simulink model "CAVE_MachE_speedTrack0202"  (R2019b)
settings: configuration reference "ConfigSetDesktopFixedStep" (kept outside this file)
PreLoadFcn:
  | VSS_BICYCLE=Simulink.Variant('Dual=0');
  | VSS_DUAL=Simulink.Variant('Dual=1');
  | Dual=1;
  | load('DriveCycle2.mat')
PostLoadFcn:
  | if any(exist('dsrtsu_mdlpostloadfcn', 'file') ~= 0), dsrtsu_mdlpostloadfcn('Execute', bdroot); end
InitFcn:
  | , if any(exist('dsmpb_private', 'file') ~= 0), dsmpb_private('dsmpb_mdlclblib', 'Init', bdroot); end,
  | load('DriveCycle2.mat')
model workspace (MAT data in the model file):
  Gas = 0.383333333333
values from neighbouring files (symbols this model uses):
  CoastDown =     [Run_Simulink.mat]
  limitedMCT =     [Run_Simulink.mat]
  MCT =     [Run_Simulink.mat]
  pMCT =     [Run_Simulink.mat]
  Ref_speed = [13 13.007895099 13.015778396 13.023649891 13.031509584 13.039357475 13.047193564 13.055017851 13.062830336 13.070631019 13.0784199 13.086196979 ... (2669 elements, 2669x1)]    [Ref_speed_and_time.mat]
  Ref_time = [0 0.01 0.02 0.03 0.04 0.05 0.06 0.07 0.08 0.09 0.1 0.11 ... (2669 elements, 2669x1)]    [Ref_speed_and_time.mat]
  US06 =     [Run_Simulink.mat]
undefined symbols (not defined in the file or in its folder): AccelCmd, ActTqLF_Nm_, ActTqLR_Nm_, ActTqRF_Nm_, ActTqRR_Nm_, BattChargeLimitMaxPwr, BattChargeLimitSocBpts, BattChargeLimitTbl, BattChrgCapcty, BattDischargeLimitSocBpts, BattDischargeLimitTbl, BattDischargeMaxPwr, BattNumCellsParallel, BattNumCellsSeries, BattOpenVoltCapBpts, BattOpenVoltTbl, BattResistSocBpts, BattResistTbl, BattResistTempBpts, BrakeMaxPrs, BrakeMaxTrq, ChassisDistCg2FrontAxle, ChassisDistCg2RearAxle, ChassisVehMass, CltchCmd, DecelCmd, DiffRatio, DiscIntNeverNeededParam, EnvGravCnst, EnvPrs, EnvTemp, FuelSpecificGrav, GearCmd, h, InitStates, lgSw, MtrEffSpdBpts, MtrEffTbl, MtrEffTrqBpts, MtrPwrMax, MtrTrqMax, Ref_Spd0229, Ref_Time0229, SteeringCmd, SupvsryCtrlRegenBrkCutOffTbl, SupvsryCtrlRegenSpdBpts, TestScnrioCycleNum, VEH
libraries: VSIGenLib x67, simulink x57, etargetslib x38, dsmpblib x28, vehdynlibtire x12, autolibshared x9, vehdynlibsuspension x7, vehdynlibtirecommon x7, autolibutils x5, CarMaker4SL x4, VsrLibWheel x4, autolibpowerinfoutils x3
(part 13 of 14)

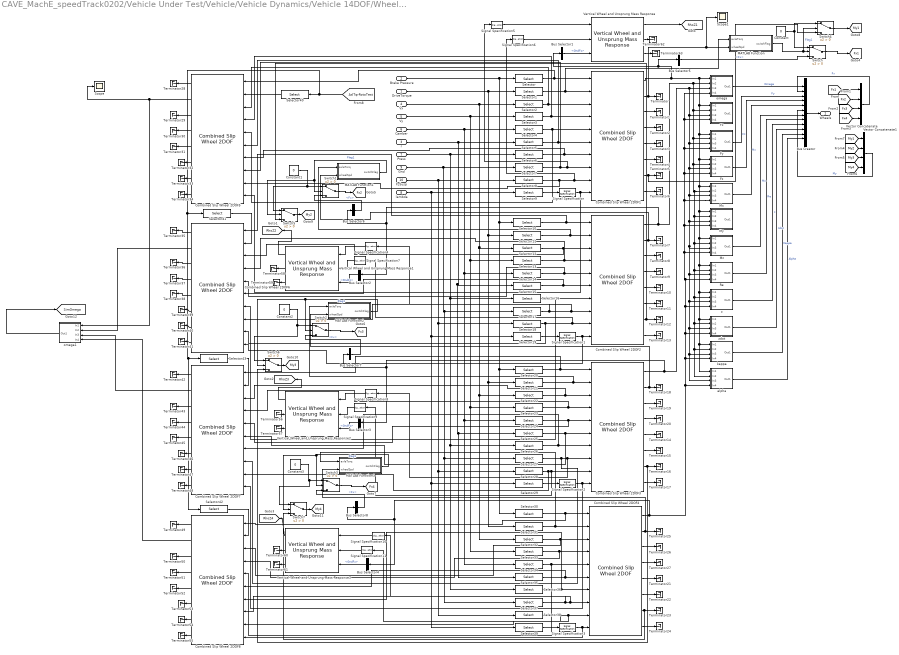
== system CAVE_MachE_speedTrack0202/Vehicle Under Test/Vehicle/Vehicle Dynamics/Vehicle 14DOF/Wheels and Tires/VDBS/Tires/MF Tires ==
  DriveTorque : Inport
  Brake Pressure : Inport  Port=2
  r : Inport  Port=3
  Vx : Inport  Port=4
  Vy : Inport  Port=5
  Camber : Inport  Port=6
  Press : Inport  Port=7  Unit=Pa
  lambda : Inport  Port=8  Unit=1
  Gnd : Inport  Port=9
  FzSusp : Inport  Port=10
  Bus Creator : BusCreator  Inputs=12
  Bus Selector{1..4} (4 alike) : BusSelector  OutputSignals=GndFz
  Bus Selector{5..8} (4 alike) : BusSelector  OutputSignals=Fx
  Combined Slip Wheel 2DOF{1..8} (8 alike) : vehdynlibtire/Combined Slip Wheel 2DOF  BrakeType=Disc  mu_static=.3  mu_kinetic=.2  disk_abore=.05  Rm=.216  num_pads=4  drum_abore=0.0508  drum_a=0.123  drum_c=0.212  drum_r=0.15  drum_theta1=0  drum_theta2=126  brake_p_bpt=[0 BrakeMaxPrs]/1e5  brake_n_bpt=[0 1000]  f_brake_t=[0 0; BrakeMaxTrq BrakeMaxTrq ]  tireParamSet=vdynPassCar.mat  plySteer=off  turnslip=off  PRESMAX=1000000  PRESMIN=10000  FZMAX=10000  FZMIN=100  VXLOW=0.1  KPUMAX=1.5  KPUMIN=-1.5  ALPMAX=1.5  ALPMIN=-1.5  CAMMAX=0.2  CAMMIN=-0.2  LONGVL=16.7  omegao=0  br=1e-3  UNLOADED_RADIUS=0.3135  NOMPRES=220000  FNOMIN=5000  WIDTH=0.235  MASS=13.37  IYY=0.82  GRAVITY=-9.81  zo=.015+0  zdoto=0  BREFF=8.25094594147963  DREFF=0.260468730454265  FREFF=0.0735298544471851  Q_RE0=1.00866439868088  Q_V1=0.000760413786224011  Q_V2=0.0463384792019201  Q_FZ1=0  Q_FZ2=15.6870832810226  Q_FZ3=0  Q_FCX=0.138643970247602  Q_FCY=0.10843499565426  Q_FCY2=-0.465763352339538  PFZ1=0.69958166705601  VERTICAL_STIFFNESS=207885.061134007  VERTICAL_DAMPING=275.3  LONGITUDINAL_STIFFNESS=388714.175879854  LATERAL_STIFFNESS=157087.404633332  PCFX1=0.18539229191199  PCFX2=0  PCFX3=0  PCFY1=0.163183345037677  PCFY2=0  PCFY3=0.249094918231954  Q_RA1=0.675942571700787  Q_RA2=0.73800463546164  Q_RB1=1.04487486456705  Q_RB2=-1.191763806629  PCX1=1.58523057950359  PDX1=1.0239116238178  PDX2=-0.0842405110022724  PDX3=0  PEX1=0.110312777158455  PEX2=0.313468516038146  PEX3=0  PEX4=0.0016060905760045  PKX1=21.3872544684023  PKX2=14.0006541873175  PKX3=-0.405326109653452  PHX1=0.000212599305364818  PHX2=0.00115950515263055  PVX1=1.59236164471432e-05  PVX2=0.000104321112127671  PPX1=-0.349461321276586  PPX2=0.387840040616429  PPX3=-0.0969947336569324  PPX4=0.0632271859795801  RBX1=12.7633329850276  RBX2=9.5787123658471  RBX3=0  RCX1=1.02796280922059  REX1=-0.45202516851367  REX2=-0.47304886171176  RHX1=0.000233272373115809  QSX1=-0.00788307788961443  QSX2=0.954629515459396  QSX3=0.0155855777667025  QSX4=0.125904607142414  QSX5=1.01110069703963  QSX6=20.1938577118433  QSX7=0.310818120717083  QSX8=-0.0430823751139655  QSX9=0.636494404888216  QSX10=0.142438060591663  QSX11=0.346766530036373  QSX12=0  QSX13=0  QSX14=0  PPMX1=0  PCY1=1.34299950037631  PDY1=0.878267729082195  PDY2=-0.0644597923147385  PDY3=0  PEY1=-0.809776534470972  PEY2=-0.600180598867198  PEY3=0.0991732552633487  PEY4=-6.5577974035573  PEY5=0  PKY1=-15.57  PKY2=1.73126522291751  PKY3=0.365349873517229  PKY4=1.98176755955416  PKY5=0  PKY6=-0.884005199550313  PKY7=-0.237259727611847  PHY1=-0.00183370557235628  PHY2=0.00346401302716671  PVY1=-0.00675427560163264  PVY2=0.036379218103843  PVY3=-0.163543984089166  PVY4=-0.491003349625726  PPY1=-0.62059646553185  PPY2=-0.0647824842338686  PPY3=-0.164648843290686  PPY4=0.283193909060098  PPY5=0  RBY1=10.7588809173639  RBY2=7.70420065295029  RBY3=3.40283755070691e-06  RBY4=0  RCY1=1.06691874059059  REY1=0.308244924574305  REY2=7.48775032604508e-06  RHY1=0.0118479204960415  RHY2=7.63650177161071e-06  RVY1=0.0560024425050078  RVY2=7.48487127056197e-06  RVY3=0  RVY4=98.4047026517149  RVY5=2.02759273900054  RVY6=15.7623064923347  QSY1=0.00699077564863536  QSY2=0  QSY3=0.00153535478298811  QSY4=8.55710322455322e-05  QSY5=0  QSY6=0  QSY7=0.89443879773793  QSY8=-0.403227641260894  QBZ1=11.666656027484  QBZ2=-1.30355438574485  QBZ3=0  QBZ4=0.177918305399071  QBZ5=-0.162481135068033  QBZ6=0  QBZ9=30.1445534682089  QBZ10=0  QCZ1=1.29026978207574  QDZ1=0.0886972644991399  QDZ2=-0.0058634820161856  QDZ3=0.3805597481383  QDZ4=0  QDZ6=0.00160914918118959  QDZ7=-0.00211036330862154  QDZ8=-0.13921904912557  QDZ9=0.00816585550028243  QDZ10=0  QDZ11=0  QEZ1=-2.19802254534746  QEZ2=1.01850535789165  QEZ3=0  QEZ4=0.278379679112054  QEZ5=-0.548414722765386  QHZ1=0.00148361198869669  QHZ2=0.00202017567585904  QHZ3=0.240316641332066  QHZ4=-0.210114035738085  PPZ1=-0.443927982388615  PPZ2=0  SSZ1=0.00914999585397887  SSZ2=0.0389830656052735  SSZ3=0  SSZ4=0  PDXP1=0.396718274678791  PDXP2=0  PDXP3=0  PKYP1=1.00587060633573  PDYP1=0.40483048923438  PDYP2=0  PDYP3=0  PDYP4=0  PHYP1=0.992731942067188  PHYP2=0.150352945499914  PHYP3=0  PHYP4=-3.98988682633674  PECP1=0.502379254513503  PECP2=0  QDTP1=10.0178654287947  QCRP1=0.200627747200702  QCRP2=0.0995735881599772  QBRP1=0.0997107127960717  QDRP1=1.01432910167423  QDRP2=0  aMode=2
      settings: SourceProductName=Vehicle Dynamics Blockset  SourceProductBaseCode=VE
  Constant{,1..3} (4 alike) : Constant  Value=0
  Fx : Subsystem
  Fy : Subsystem
  Fz : Subsystem
  MATLAB Function : MATLAB Function  TreatAsAtomicUnit=on
  MATLAB Function1 : MATLAB Function  TreatAsAtomicUnit=on
  MATLAB Function2 : MATLAB Function  TreatAsAtomicUnit=on
  MATLAB Function3 : MATLAB Function  TreatAsAtomicUnit=on
  Mx : Subsystem
  My : Subsystem
  Mz : Subsystem
  Re : Subsystem
  Scope : Scope
  Scope1 : Scope
  Selector{,1..8,40} (10 alike) : Selector  InputPortWidth=4  IndexOptions=Index vector (dialog)  Indices=1  OutputSizes=1
  Selector{10..18,41} (10 alike) : Selector  InputPortWidth=4  IndexOptions=Index vector (dialog)  Indices=2  OutputSizes=1
  Selector19 : Selector  NumberOfDimensions=2  InputPortWidth=4  IndexOptions=Select all,Index vector (dialog)  Indices=1,2  OutputSizes=1,1
  Selector{20..28,43} (10 alike) : Selector  InputPortWidth=4  IndexOptions=Index vector (dialog)  Indices=3  OutputSizes=1
  Selector29 : Selector  NumberOfDimensions=2  InputPortWidth=4  IndexOptions=Select all,Index vector (dialog)  Indices=1,3  OutputSizes=1,1
  Selector{30..38,42} (10 alike) : Selector  InputPortWidth=4  IndexOptions=Index vector (dialog)  Indices=4  OutputSizes=1
  Selector39 : Selector  NumberOfDimensions=2  InputPortWidth=4  IndexOptions=Select all,Index vector (dialog)  Indices=1,4  OutputSizes=1,1
  Selector9 : Selector  NumberOfDimensions=2  InputPortWidth=4  IndexOptions=Select all,Index vector (dialog)  Indices=1,1  OutputSizes=1,1
  Signal Specification{,1..3} (4 alike) : SignalSpecification  Unit=1
  Signal Specification{4..5,8,10} (4 alike) : SignalSpecification  Unit=m
  Signal Specification{6..7,9,11} (4 alike) : SignalSpecification  Unit=N
  Switch{,1..7} (8 alike) : Switch  Criteria=u2 > Threshold
  Terminator{,1..63} (64 alike) : Terminator
  Vector Concatenate : Concatenate  NumInputs=4
  Vector Concatenate1 : Concatenate  NumInputs=4
  Vertical Wheel and Unsprung Mass Response{,1..3} (4 alike) : vehdynlibtirecommon/Vertical Wheel and Unsprung Mass Response  m=13.37  bz=275.3  zo=0.015  zdoto=0  g=-9.81  ReMax=0.3135
      settings: SourceProductName=Vehicle Dynamics Blockset  SourceProductBaseCode=VE
  alpha : Subsystem
  kappa : Subsystem
  omega : Subsystem
  omega1 : Subsystem
  z : Subsystem
  zdot : Subsystem
  Wheels : Outport  VectorParamsAs1DForOutWhenUnconnected=off
  tag scope: Fx1=global, Fx2=global, Fx3=global, Fx4=global, My1=global, My2=global, My3=global, My4=global, RhoZ1=global, RhoZ2=global, RhoZ3=global, RhoZ4=global, SimOmega=global
  wires:
  Bus Creator/1 -> Wheels/1
  Brake Pressure/1 -> Selector30/1, Selector20/1, Selector10/1, Selector/1
  DriveTorque/1 -> Selector31/1, Selector21/1, Selector11/1, Selector1/1
  Vx/1 -> Selector12/1, Selector32/1, Selector22/1, Selector2/1
  Selector/1 -> Combined Slip Wheel 2DOF5/1, Combined Slip Wheel 2DOF1/1
  Selector1/1 -> MATLAB Function/1(axleTorq), Combined Slip Wheel 2DOF1/2
  Selector7/1 -> Combined Slip Wheel 2DOF5/8, Signal Specification5/1, Combined Slip Wheel 2DOF1/8
  Selector6/1 -> Combined Slip Wheel 2DOF5/7, Combined Slip Wheel 2DOF1/7
  Selector5/1 -> Combined Slip Wheel 2DOF5/6, Combined Slip Wheel 2DOF1/6
  Selector4/1 -> Combined Slip Wheel 2DOF5/5, Combined Slip Wheel 2DOF1/5
  Selector9/1 -> Signal Specification/1
  Selector8/1 -> Combined Slip Wheel 2DOF5/9, Signal Specification6/1, Combined Slip Wheel 2DOF1/9
  Camber/1 -> Selector34/1, Selector24/1, Selector14/1, Selector4/1
  Vy/1 -> Selector33/1, Selector23/1, Selector13/1, Selector3/1
  r/1 -> Selector15/1, Selector35/1, Selector25/1, Selector5/1
  Press/1 -> Selector36/1, Selector26/1, Selector16/1, Selector6/1
  Gnd/1 -> Selector37/1, Selector27/1, Selector17/1, Selector7/1
  FzSusp/1 -> Selector38/1, Selector28/1, Selector18/1, Selector8/1
  lambda/1 -> Selector9/1, Selector19/1, Selector39/1, Selector29/1
  Selector18/1 -> Combined Slip Wheel 2DOF6/9, Signal Specification7/1, Combined Slip Wheel 2DOF2/9
  Selector19/1 -> Signal Specification1/1
  Selector14/1 -> Combined Slip Wheel 2DOF6/5, Combined Slip Wheel 2DOF2/5
  Selector15/1 -> Combined Slip Wheel 2DOF6/6, Combined Slip Wheel 2DOF2/6
  Selector16/1 -> Combined Slip Wheel 2DOF6/7, Combined Slip Wheel 2DOF2/7
  Selector17/1 -> Combined Slip Wheel 2DOF6/8, Signal Specification4/1, Combined Slip Wheel 2DOF2/8
  Selector12/1 -> Combined Slip Wheel 2DOF6/3, Combined Slip Wheel 2DOF2/3
  Selector13/1 -> Combined Slip Wheel 2DOF6/4, Combined Slip Wheel 2DOF2/4
  Selector11/1 -> MATLAB Function1/1(axleTorq), Combined Slip Wheel 2DOF2/2
  Selector10/1 -> Combined Slip Wheel 2DOF6/1, Combined Slip Wheel 2DOF2/1
  Selector30/1 -> Combined Slip Wheel 2DOF8/1, Combined Slip Wheel 2DOF4/1
  Selector33/1 -> Combined Slip Wheel 2DOF8/4, Combined Slip Wheel 2DOF4/4
  Selector32/1 -> Combined Slip Wheel 2DOF8/3, Combined Slip Wheel 2DOF4/3
  Selector37/1 -> Signal Specification10/1, Combined Slip Wheel 2DOF8/8, Combined Slip Wheel 2DOF4/8
  Selector36/1 -> Combined Slip Wheel 2DOF8/7, Combined Slip Wheel 2DOF4/7
  Selector35/1 -> Combined Slip Wheel 2DOF8/6, Combined Slip Wheel 2DOF4/6
  Selector34/1 -> Combined Slip Wheel 2DOF4/5, Combined Slip Wheel 2DOF8/5
  Selector39/1 -> Signal Specification3/1
  Selector29/1 -> Signal Specification2/1
  Selector24/1 -> Combined Slip Wheel 2DOF7/5, Combined Slip Wheel 2DOF3/5
  Selector25/1 -> Combined Slip Wheel 2DOF7/6, Combined Slip Wheel 2DOF3/6
  Selector26/1 -> Combined Slip Wheel 2DOF7/7, Combined Slip Wheel 2DOF3/7
  Selector22/1 -> Combined Slip Wheel 2DOF7/3, Combined Slip Wheel 2DOF3/3
  Selector23/1 -> Combined Slip Wheel 2DOF7/4, Combined Slip Wheel 2DOF3/4
  Selector20/1 -> Combined Slip Wheel 2DOF7/1, Combined Slip Wheel 2DOF3/1
  Combined Slip Wheel 2DOF1/1 -> Bus Selector5/1, Bus Selector1/1, Mx/1(In1), My/1(In1), alpha/1(In1), kappa/1(In1), zdot/1(In1), z/1(In1), Re/1(In1), Mz/1(In1), Fz/1(In1), Fy/1(In1), Fx/1(In1), omega/1(In1)
  omega/1(Out1) -> Bus Creator/1  "Omega"
  Mz/1(Out1) -> Bus Creator/7  "Mz"
  Fz/1(Out1) -> Bus Creator/4  "Fz"
  Re/1(Out1) -> Bus Creator/8  "Re"
  z/1(Out1) -> Bus Creator/9  "z"
  zdot/1(Out1) -> Bus Creator/10  "zdot"
  Mx/1(Out1) -> Bus Creator/5  "Mx"
  kappa/1(Out1) -> Bus Creator/11  "Kappa"
  Fy/1(Out1) -> Bus Creator/3  "Fy"
  Selector2/1 -> Combined Slip Wheel 2DOF5/3, Combined Slip Wheel 2DOF1/3
  Selector3/1 -> Combined Slip Wheel 2DOF5/4, Combined Slip Wheel 2DOF1/4
  Signal Specification/1 -> Combined Slip Wheel 2DOF5/10, Combined Slip Wheel 2DOF1/10
  Signal Specification1/1 -> Combined Slip Wheel 2DOF6/10, Combined Slip Wheel 2DOF2/10
  Signal Specification2/1 -> Combined Slip Wheel 2DOF7/10, Combined Slip Wheel 2DOF3/10
  Signal Specification3/1 -> Combined Slip Wheel 2DOF8/10, Combined Slip Wheel 2DOF4/10
  Combined Slip Wheel 2DOF1/2 -> Scope1/1, MATLAB Function/2(wheelSpd), Terminator/1
  Combined Slip Wheel 2DOF1/3 -> Terminator1/1
  Combined Slip Wheel 2DOF1/4 -> Terminator2/1
  Combined Slip Wheel 2DOF1/7 -> Switch4/3, Terminator5/1
  Combined Slip Wheel 2DOF1/6 -> Terminator4/1
  Combined Slip Wheel 2DOF1/5 -> Terminator3/1
  Combined Slip Wheel 2DOF1/8 -> Terminator6/1
  Combined Slip Wheel 2DOF2/2 -> MATLAB Function1/2(wheelSpd), Terminator7/1
  Combined Slip Wheel 2DOF2/3 -> Terminator8/1
  Combined Slip Wheel 2DOF2/4 -> Terminator9/1
  Combined Slip Wheel 2DOF2/5 -> Terminator10/1
  Combined Slip Wheel 2DOF2/6 -> Terminator11/1
  Combined Slip Wheel 2DOF2/7 -> Switch5/3, Terminator12/1
  Combined Slip Wheel 2DOF2/8 -> Terminator13/1
  Combined Slip Wheel 2DOF3/3 -> Terminator19/1
  Combined Slip Wheel 2DOF3/4 -> Terminator20/1
  Combined Slip Wheel 2DOF3/5 -> Terminator14/1
  Combined Slip Wheel 2DOF3/6 -> Terminator15/1
  Combined Slip Wheel 2DOF3/7 -> Switch6/3, Terminator16/1
  Combined Slip Wheel 2DOF3/8 -> Terminator17/1
  Combined Slip Wheel 2DOF4/3 -> Terminator26/1
  Combined Slip Wheel 2DOF4/4 -> Terminator27/1
  Combined Slip Wheel 2DOF4/5 -> Terminator21/1
  Combined Slip Wheel 2DOF4/6 -> Terminator22/1
  Combined Slip Wheel 2DOF4/7 -> Switch7/3, Terminator23/1
  Combined Slip Wheel 2DOF4/8 -> Terminator24/1
  alpha/1(Out1) -> Bus Creator/12  "Alpha"
  Signal Specification5/1 -> Vertical Wheel and Unsprung Mass Response/1
  Signal Specification6/1 -> Vertical Wheel and Unsprung Mass Response/2
  Bus Selector1/1 -> Vertical Wheel and Unsprung Mass Response/3  "<GndFz>"
  Vertical Wheel and Unsprung Mass Response/1 -> [RhoZ1]
  Bus Selector2/1 -> Vertical Wheel and Unsprung Mass Response1/3  "<GndFz>"
  Signal Specification7/1 -> Vertical Wheel and Unsprung Mass Response1/2
  Vertical Wheel and Unsprung Mass Response1/1 -> [RhoZ2]
  Signal Specification4/1 -> Vertical Wheel and Unsprung Mass Response1/1
  Bus Selector3/1 -> Vertical Wheel and Unsprung Mass Response2/3  "<GndFz>"
  Signal Specification9/1 -> Vertical Wheel and Unsprung Mass Response2/2
  Selector28/1 -> Combined Slip Wheel 2DOF3/9, Signal Specification9/1, Combined Slip Wheel 2DOF7/9
  Vertical Wheel and Unsprung Mass Response2/1 -> [RhoZ3]
  Signal Specification8/1 -> Vertical Wheel and Unsprung Mass Response2/1
  Combined Slip Wheel 2DOF3/1 -> My/3(In3), alpha/3(In3), kappa/3(In3), zdot/3(In3), z/3(In3), Re/3(In3), Mz/3(In3), Mx/3(In3), Fz/3(In3), Fy/3(In3), Fx/3(In3), omega/3(In3), Bus Selector3/1, Bus Selector7/1
  Selector38/1 -> Signal Specification11/1, Combined Slip Wheel 2DOF8/9, Combined Slip Wheel 2DOF4/9
  Signal Specification11/1 -> Vertical Wheel and Unsprung Mass Response3/2
  Signal Specification10/1 -> Vertical Wheel and Unsprung Mass Response3/1
  Combined Slip Wheel 2DOF4/1 -> omega/4(In4), Fx/4(In4), Fy/4(In4), Fz/4(In4), Mx/4(In4), My/4(In4), Mz/4(In4), Re/4(In4), z/4(In4), zdot/4(In4), kappa/4(In4), alpha/4(In4), Bus Selector8/1, Bus Selector4/1
  Vertical Wheel and Unsprung Mass Response3/1 -> [RhoZ4]
  Bus Selector4/1 -> Vertical Wheel and Unsprung Mass Response3/3  "<GndFz>"
  Bus Selector5/1 -> Switch/3  "<Fx>"
  Combined Slip Wheel 2DOF2/1 -> Bus Selector2/1, Bus Selector6/1, omega/2(In2), Fx/2(In2), Mx/2(In2), My/2(In2), alpha/2(In2), kappa/2(In2), zdot/2(In2), z/2(In2), Re/2(In2), Mz/2(In2), Fz/2(In2), Fy/2(In2)
  Constant/1 -> Switch4/1, Switch/1
  MATLAB Function/1(switchFlag) -> Switch4/2, Switch/2  "Flag1"
  Switch/1 -> [Fx1]
  Constant1/1 -> Switch1/1, Switch5/1
  Switch1/1 -> [Fx2]
  MATLAB Function1/1(switchFlag) -> Switch5/2, Switch1/2  "Flag1"
  Bus Selector6/1 -> Switch1/3  "<Fx>"
  Switch2/1 -> [Fx3]
  MATLAB Function2/1(switchFlag) -> Switch6/2, Switch2/2  "Flag1"
  Selector21/1 -> MATLAB Function2/1(axleTorq), Combined Slip Wheel 2DOF3/2
  Combined Slip Wheel 2DOF3/2 -> Terminator18/1, MATLAB Function2/2(wheelSpd)
  Bus Selector7/1 -> Switch2/3  "<Fx>"
  Constant2/1 -> Switch6/1, Switch2/1
  Switch3/1 -> [Fx4]
  MATLAB Function3/1(switchFlag) -> Switch7/2, Switch3/2  "Flag1"
  Selector31/1 -> Combined Slip Wheel 2DOF4/2, MATLAB Function3/1(axleTorq)
  Combined Slip Wheel 2DOF4/2 -> Terminator25/1, MATLAB Function3/2(wheelSpd)
  Bus Selector8/1 -> Switch3/3  "<Fx>"
  Constant3/1 -> Switch7/1, Switch3/1
  [Fx1] -> Vector Concatenate/1
  [Fx2] -> Vector Concatenate/2
  [Fx3] -> Vector Concatenate/3
  [Fx4] -> Vector Concatenate/4
  Vector Concatenate/1 -> Bus Creator/2  "Fx"
  Switch4/1 -> [My1]
  Switch5/1 -> [My2]
  Switch6/1 -> [My3]
  Switch7/1 -> [My4]
  [My1] -> Vector Concatenate1/1
  [My2] -> Vector Concatenate1/2
  [My3] -> Vector Concatenate1/3
  [My4] -> Vector Concatenate1/4
  Vector Concatenate1/1 -> Bus Creator/6  "My"
  [AxlTqrRotoTest] -> Selector42/1, Selector43/1, Selector41/1, Selector40/1
  Selector40/1 -> Combined Slip Wheel 2DOF5/2
  Combined Slip Wheel 2DOF5/1 -> Terminator28/1
  Combined Slip Wheel 2DOF5/3 -> Terminator29/1
  Combined Slip Wheel 2DOF5/4 -> Terminator30/1
  Combined Slip Wheel 2DOF5/5 -> Terminator31/1
  Combined Slip Wheel 2DOF5/6 -> Terminator32/1
  Combined Slip Wheel 2DOF5/7 -> Terminator33/1
  Combined Slip Wheel 2DOF5/8 -> Terminator34/1
  Combined Slip Wheel 2DOF6/8 -> Terminator41/1
  Combined Slip Wheel 2DOF6/7 -> Terminator40/1
  Combined Slip Wheel 2DOF6/6 -> Terminator39/1
  Combined Slip Wheel 2DOF6/1 -> Terminator35/1
  Combined Slip Wheel 2DOF6/3 -> Terminator36/1
  Combined Slip Wheel 2DOF6/4 -> Terminator37/1
  Combined Slip Wheel 2DOF6/5 -> Terminator38/1
  Selector41/1 -> Combined Slip Wheel 2DOF6/2
  Combined Slip Wheel 2DOF7/5 -> Terminator45/1
  Combined Slip Wheel 2DOF7/4 -> Terminator44/1
  Combined Slip Wheel 2DOF7/3 -> Terminator43/1
  Combined Slip Wheel 2DOF7/1 -> Terminator42/1
  Combined Slip Wheel 2DOF7/6 -> Terminator46/1
  Combined Slip Wheel 2DOF7/7 -> Terminator47/1
  Combined Slip Wheel 2DOF7/8 -> Terminator48/1
  Selector27/1 -> Combined Slip Wheel 2DOF7/8, Signal Specification8/1, Combined Slip Wheel 2DOF3/8
  Combined Slip Wheel 2DOF8/7 -> Terminator54/1
  Combined Slip Wheel 2DOF8/4 -> Terminator51/1
  Combined Slip Wheel 2DOF8/1 -> Terminator49/1
  Combined Slip Wheel 2DOF8/3 -> Terminator50/1
  Combined Slip Wheel 2DOF8/5 -> Terminator52/1
  Combined Slip Wheel 2DOF8/6 -> Terminator53/1
  Combined Slip Wheel 2DOF8/8 -> Terminator55/1
  Selector43/1 -> Combined Slip Wheel 2DOF7/2
  Selector42/1 -> Combined Slip Wheel 2DOF8/2
  Combined Slip Wheel 2DOF5/2 -> omega1/1(In1), Scope/1
  Combined Slip Wheel 2DOF6/2 -> omega1/2(In2)
  Combined Slip Wheel 2DOF7/2 -> omega1/3(In3)
  Combined Slip Wheel 2DOF8/2 -> omega1/4(In4)
  omega1/1(Out1) -> [SimOmega]
  Vertical Wheel and Unsprung Mass Response2/2 -> Terminator56/1
  Vertical Wheel and Unsprung Mass Response2/3 -> Terminator57/1
  Vertical Wheel and Unsprung Mass Response1/2 -> Terminator58/1
  Vertical Wheel and Unsprung Mass Response1/3 -> Terminator59/1
  Vertical Wheel and Unsprung Mass Response3/2 -> Terminator60/1
  Vertical Wheel and Unsprung Mass Response3/3 -> Terminator61/1
  Vertical Wheel and Unsprung Mass Response/2 -> Terminator62/1
  Vertical Wheel and Unsprung Mass Response/3 -> Terminator63/1

== system CAVE_MachE_speedTrack0202/Vehicle Under Test/Vehicle/Vehicle Dynamics/Vehicle 14DOF/Wheels and Tires/VDBS/Veh2Tire/Wheel Angles ==
  steer : Inport
  camber : Inport  Port=2
  Add1 : Sum
  Add2 : Sum
  Constant1 : Constant  Value=pi
  Constant2 : Constant  Value=[pi;0;pi;0].*0+[0;pi;0;pi].*0
  Constant3 : Constant  Value=ones(1,4).*0
  Reshape : Reshape  OutputDimensionality=Row vector (2-D)
  Reshape1 : Reshape  OutputDimensionality=Row vector (2-D)
  Reshape2 : Reshape  OutputDimensionality=Row vector (2-D)
  Vector Concatenate3 : Concatenate  NumInputs=3  Mode=Multidimensional array
  Vehicle : Outport  VectorParamsAs1DForOutWhenUnconnected=off
  wires:
  Constant2/1 -> Add1/2
  Constant3/1 -> Reshape2/1
  Vector Concatenate3/1 -> Vehicle/1
  Reshape/1 -> Vector Concatenate3/3
  Reshape1/1 -> Vector Concatenate3/1
  camber/1 -> Add2/1
  Reshape2/1 -> Vector Concatenate3/2
  steer/1 -> Add1/1
  Add1/1 -> Reshape/1
  Constant1/1 -> Add2/2
  Add2/1 -> Reshape1/1

== system CAVE_MachE_speedTrack0202/Vehicle Under Test/Vehicle/Vehicle Dynamics/Vehicle 14DOF/Wheels and Tires/VDBS/Veh2Tire/Wheel to Body Transform ==
  VelVeh : Inport  Partition=on  PartitionDimension=2  PartitionWidth=1  PartitionOffset=0
  WheelAngles : Inport  Port=2  Partition=on  PartitionDimension=2  PartitionWidth=1  PartitionOffset=0
  Demux1 : Demux  Outputs=3
  Divide1 : Product  Inputs=**  Multiplication=Matrix(*)
  For Each : ForEach  DisableCoverage=on
  Rotation Angles to Direction Cosine Matrix : sharedtransform/Rotation Angles to Direction Cosine Matrix  rotationOrder=ZYX  aMode=2
      settings: SourceProductBaseCode=AE
  Selector : Selector  InputPortWidth=3  IndexOptions=Index vector (dialog)  Indices=[3 2 1]  OutputSizes=1
  xdotWheel : Outport  ConcatenationDimension=1  VectorParamsAs1DForOutWhenUnconnected=off
  ydotWheel : Outport  Port=2  ConcatenationDimension=1  VectorParamsAs1DForOutWhenUnconnected=off
  zdotWheel : Outport  Port=3  ConcatenationDimension=1  VectorParamsAs1DForOutWhenUnconnected=off
  wires:
  Divide1/1 -> Demux1/1
  Demux1/1 -> xdotWheel/1
  Demux1/2 -> ydotWheel/1
  Demux1/3 -> zdotWheel/1
  Rotation Angles to Direction Cosine Matrix/1 -> Divide1/1
  VelVeh/1 -> Divide1/2
  WheelAngles/1 -> Selector/1
  Selector/1 -> Rotation Angles to Direction Cosine Matrix/1

== system CAVE_MachE_speedTrack0202/Vehicle Under Test/Vehicle/Vehicle Dynamics/Vehicle 7DOF/Longitudinal Wheels 4DOF/Velocity and Vertical Load/Bicycle/Bicycle Fz ==
  In1 : Inport
  Bus Selector6 : BusSelector  OutputSignals=BdyFrm.Forces.Tires.FrntTire.Fz,BdyFrm.Forces.Tires.RearTire.Fz
  Cont LPF : autolibutils/Cont LPF  wc=20*2*pi  aMode=2
      settings: SourceProductName=Powertrain Blockset  SourceProductBaseCode=PW
  Mux5 : Mux
  Saturation : Saturate  UpperLimit=20e3  LowerLimit=1000  ZeroCross=off
  Out1 : Outport  VectorParamsAs1DForOutWhenUnconnected=off
  wires:
  Cont LPF/1 -> Out1/1
  Saturation/1 -> Cont LPF/1
  Bus Selector6/2 -> Mux5/4, Mux5/3  "<Fz>"
  In1/1 -> Bus Selector6/1
  Bus Selector6/1 -> Mux5/2, Mux5/1  "<Fz>"
  Mux5/1 -> Saturation/1

== system CAVE_MachE_speedTrack0202/Vehicle Under Test/Vehicle/Vehicle Dynamics/Vehicle 7DOF/Longitudinal Wheels 4DOF/Velocity and Vertical Load/Bicycle/Bicycle V ==
  In1 : Inport
  Bus Selector : BusSelector  OutputSignals=BdyFrm.FrntAxl.Vel.xdot,BdyFrm.FrntAxl.Vel.ydot,BdyFrm.FrntAxl.Vel.zdot  OutputAsBus=on
  Bus Selector3 : BusSelector  OutputSignals=BdyFrm.RearAxl.Vel.xdot,BdyFrm.RearAxl.Vel.ydot,BdyFrm.RearAxl.Vel.zdot  OutputAsBus=on
  Bus to Vector1 : BusToVector
  Bus to Vector3 : BusToVector
  Vector Concatenate1 : Concatenate  NumInputs=4  Mode=Multidimensional array  ConcatenateDimension=2
  Out1 : Outport  VectorParamsAs1DForOutWhenUnconnected=off
  wires:
  Bus Selector3/1 -> Bus to Vector3/1
  Bus to Vector1/1 -> Vector Concatenate1/2, Vector Concatenate1/1
  In1/1 -> Bus Selector3/1, Bus Selector/1
  Bus Selector/1 -> Bus to Vector1/1
  Bus to Vector3/1 -> Vector Concatenate1/4, Vector Concatenate1/3
  Vector Concatenate1/1 -> Out1/1

== system CAVE_MachE_speedTrack0202/Vehicle Under Test/Vehicle/Vehicle Dynamics/Vehicle 7DOF/Longitudinal Wheels 4DOF/Velocity and Vertical Load/Dual/Dual Fz ==
  In1 : Inport
  Bus Selector6 : BusSelector  OutputSignals=BdyFrm.Forces.Tires.FrntTires.Lft.Fz,BdyFrm.Forces.Tires.FrntTires.Rght.Fz,BdyFrm.Forces.Tires.RearTires.Lft.Fz,BdyFrm.Forces.Tires.RearTires.Rght.Fz
  Cont LPF : autolibutils/Cont LPF  wc=20*2*pi  aMode=2
      settings: SourceProductName=Powertrain Blockset  SourceProductBaseCode=PW
  Saturation : Saturate  UpperLimit=20e3  LowerLimit=1000  ZeroCross=off
  Vector Concatenate : Concatenate  NumInputs=4
  Out1 : Outport  VectorParamsAs1DForOutWhenUnconnected=off
  wires:
  In1/1 -> Bus Selector6/1
  Saturation/1 -> Cont LPF/1
  Cont LPF/1 -> Out1/1
  Vector Concatenate/1 -> Saturation/1
  Bus Selector6/2 -> Vector Concatenate/2  "<Fz>"
  Bus Selector6/1 -> Vector Concatenate/1  "<Fz>"
  Bus Selector6/3 -> Vector Concatenate/3  "<Fz>"
  Bus Selector6/4 -> Vector Concatenate/4  "<Fz>"

== system CAVE_MachE_speedTrack0202/Vehicle Under Test/Vehicle/Vehicle Dynamics/Vehicle 7DOF/Longitudinal Wheels 4DOF/Velocity and Vertical Load/Dual/Dual V ==
  In1 : Inport
  Bus Selector1 : BusSelector  OutputSignals=BdyFrm.FrntAxl.Lft.Vel.xdot,BdyFrm.FrntAxl.Lft.Vel.ydot,BdyFrm.FrntAxl.Lft.Vel.zdot  OutputAsBus=on
  Bus Selector2 : BusSelector  OutputSignals=BdyFrm.FrntAxl.Rght.Vel.xdot,BdyFrm.FrntAxl.Rght.Vel.ydot,BdyFrm.FrntAxl.Rght.Vel.zdot  OutputAsBus=on
  Bus Selector4 : BusSelector  OutputSignals=BdyFrm.RearAxl.Lft.Vel.xdot,BdyFrm.RearAxl.Lft.Vel.ydot,BdyFrm.RearAxl.Lft.Vel.zdot  OutputAsBus=on
  Bus Selector5 : BusSelector  OutputSignals=BdyFrm.RearAxl.Rght.Vel.xdot,BdyFrm.RearAxl.Rght.Vel.ydot,BdyFrm.RearAxl.Rght.Vel.zdot  OutputAsBus=on
  Bus to Vector{5..8} (4 alike) : BusToVector
  Vector Concatenate2 : Concatenate  NumInputs=4  Mode=Multidimensional array  ConcatenateDimension=2
  Out1 : Outport  VectorParamsAs1DForOutWhenUnconnected=off
  wires:
  Bus to Vector6/1 -> Vector Concatenate2/2
  Bus Selector2/1 -> Bus to Vector6/1
  Bus to Vector8/1 -> Vector Concatenate2/4
  Bus Selector4/1 -> Bus to Vector7/1
  Bus to Vector5/1 -> Vector Concatenate2/1
  Bus Selector1/1 -> Bus to Vector5/1
  In1/1 -> Bus Selector1/1, Bus Selector2/1, Bus Selector4/1, Bus Selector5/1
  Bus Selector5/1 -> Bus to Vector8/1
  Bus to Vector7/1 -> Vector Concatenate2/3
  Vector Concatenate2/1 -> Out1/1

== system CAVE_MachE_speedTrack0202/Vehicle Under Test/Vehicle/Vehicle Dynamics/Vehicle 14DOF/Wheels and Tires/VDBS/Tires/Fiala Tires/Fx ==
  In1 : Inport
  In2 : Inport  Port=2
  In3 : Inport  Port=3
  In4 : Inport  Port=4
  Bus Selector{,1..3} (4 alike) : BusSelector  OutputSignals=Fx
  Vector Concatenate : Concatenate  NumInputs=4
  Out1 : Outport  VectorParamsAs1DForOutWhenUnconnected=off
  wires:
  Bus Selector3/1 -> Vector Concatenate/4  "<Fx>"
  Bus Selector2/1 -> Vector Concatenate/3  "<Fx>"
  Bus Selector1/1 -> Vector Concatenate/2  "<Fx>"
  In4/1 -> Bus Selector3/1
  In3/1 -> Bus Selector2/1
  In2/1 -> Bus Selector1/1
  Bus Selector/1 -> Vector Concatenate/1  "<Fx>"
  In1/1 -> Bus Selector/1
  Vector Concatenate/1 -> Out1/1

== system CAVE_MachE_speedTrack0202/Vehicle Under Test/Vehicle/Vehicle Dynamics/Vehicle 14DOF/Wheels and Tires/VDBS/Tires/Fiala Tires/Fy ==
  In1 : Inport
  In2 : Inport  Port=2
  In3 : Inport  Port=3
  In4 : Inport  Port=4
  Bus Selector{,1..3} (4 alike) : BusSelector  OutputSignals=Fy
  Vector Concatenate : Concatenate  NumInputs=4
  Out1 : Outport  VectorParamsAs1DForOutWhenUnconnected=off
  wires:
  Vector Concatenate/1 -> Out1/1
  In1/1 -> Bus Selector/1
  Bus Selector/1 -> Vector Concatenate/1  "<Fy>"
  In2/1 -> Bus Selector1/1
  In3/1 -> Bus Selector2/1
  In4/1 -> Bus Selector3/1
  Bus Selector1/1 -> Vector Concatenate/2  "<Fy>"
  Bus Selector2/1 -> Vector Concatenate/3  "<Fy>"
  Bus Selector3/1 -> Vector Concatenate/4  "<Fy>"

== system CAVE_MachE_speedTrack0202/Vehicle Under Test/Vehicle/Vehicle Dynamics/Vehicle 14DOF/Wheels and Tires/VDBS/Tires/Fiala Tires/Fz ==
  In1 : Inport
  In2 : Inport  Port=2
  In3 : Inport  Port=3
  In4 : Inport  Port=4
  Bus Selector{,1..3} (4 alike) : BusSelector  OutputSignals=Fz
  Vector Concatenate : Concatenate  NumInputs=4
  Out1 : Outport  VectorParamsAs1DForOutWhenUnconnected=off
  wires:
  Vector Concatenate/1 -> Out1/1
  In1/1 -> Bus Selector/1
  Bus Selector/1 -> Vector Concatenate/1  "<Fz>"
  In2/1 -> Bus Selector1/1
  In3/1 -> Bus Selector2/1
  In4/1 -> Bus Selector3/1
  Bus Selector1/1 -> Vector Concatenate/2  "<Fz>"
  Bus Selector2/1 -> Vector Concatenate/3  "<Fz>"
  Bus Selector3/1 -> Vector Concatenate/4  "<Fz>"

== system CAVE_MachE_speedTrack0202/Vehicle Under Test/Vehicle/Vehicle Dynamics/Vehicle 14DOF/Wheels and Tires/VDBS/Tires/Fiala Tires/Mx ==
  In1 : Inport
  In2 : Inport  Port=2
  In3 : Inport  Port=3
  In4 : Inport  Port=4
  Bus Selector{,1..3} (4 alike) : BusSelector  OutputSignals=Mx
  Vector Concatenate : Concatenate  NumInputs=4
  Out1 : Outport  VectorParamsAs1DForOutWhenUnconnected=off
  wires:
  Vector Concatenate/1 -> Out1/1
  In1/1 -> Bus Selector/1
  Bus Selector/1 -> Vector Concatenate/1  "<Mx>"
  In2/1 -> Bus Selector1/1
  In3/1 -> Bus Selector2/1
  In4/1 -> Bus Selector3/1
  Bus Selector1/1 -> Vector Concatenate/2  "<Mx>"
  Bus Selector2/1 -> Vector Concatenate/3  "<Mx>"
  Bus Selector3/1 -> Vector Concatenate/4  "<Mx>"

== system CAVE_MachE_speedTrack0202/Vehicle Under Test/Vehicle/Vehicle Dynamics/Vehicle 14DOF/Wheels and Tires/VDBS/Tires/Fiala Tires/My ==
  In1 : Inport
  In2 : Inport  Port=2
  In3 : Inport  Port=3
  In4 : Inport  Port=4
  Bus Selector{,1..3} (4 alike) : BusSelector  OutputSignals=My
  Vector Concatenate : Concatenate  NumInputs=4
  Out1 : Outport  VectorParamsAs1DForOutWhenUnconnected=off
  wires:
  Bus Selector3/1 -> Vector Concatenate/4  "<My>"
  Bus Selector2/1 -> Vector Concatenate/3  "<My>"
  Bus Selector1/1 -> Vector Concatenate/2  "<My>"
  In4/1 -> Bus Selector3/1
  In3/1 -> Bus Selector2/1
  In2/1 -> Bus Selector1/1
  Bus Selector/1 -> Vector Concatenate/1  "<My>"
  In1/1 -> Bus Selector/1
  Vector Concatenate/1 -> Out1/1

== system CAVE_MachE_speedTrack0202/Vehicle Under Test/Vehicle/Vehicle Dynamics/Vehicle 14DOF/Wheels and Tires/VDBS/Tires/Fiala Tires/Mz ==
  In1 : Inport
  In2 : Inport  Port=2
  In3 : Inport  Port=3
  In4 : Inport  Port=4
  Bus Selector{,1..3} (4 alike) : BusSelector  OutputSignals=Mz
  Vector Concatenate : Concatenate  NumInputs=4
  Out1 : Outport  VectorParamsAs1DForOutWhenUnconnected=off
  wires:
  Bus Selector3/1 -> Vector Concatenate/4  "<Mz>"
  Bus Selector2/1 -> Vector Concatenate/3  "<Mz>"
  Bus Selector1/1 -> Vector Concatenate/2  "<Mz>"
  In4/1 -> Bus Selector3/1
  In3/1 -> Bus Selector2/1
  In2/1 -> Bus Selector1/1
  Bus Selector/1 -> Vector Concatenate/1  "<Mz>"
  In1/1 -> Bus Selector/1
  Vector Concatenate/1 -> Out1/1

== system CAVE_MachE_speedTrack0202/Vehicle Under Test/Vehicle/Vehicle Dynamics/Vehicle 14DOF/Wheels and Tires/VDBS/Tires/Fiala Tires/Re ==
  In1 : Inport
  In2 : Inport  Port=2
  In3 : Inport  Port=3
  In4 : Inport  Port=4
  Bus Selector{,1..3} (4 alike) : BusSelector  OutputSignals=Re
  Vector Concatenate : Concatenate  NumInputs=4
  Out1 : Outport  VectorParamsAs1DForOutWhenUnconnected=off
  wires:
  Vector Concatenate/1 -> Out1/1
  In1/1 -> Bus Selector/1
  Bus Selector/1 -> Vector Concatenate/1  "<Re>"
  In2/1 -> Bus Selector1/1
  In3/1 -> Bus Selector2/1
  In4/1 -> Bus Selector3/1
  Bus Selector1/1 -> Vector Concatenate/2  "<Re>"
  Bus Selector2/1 -> Vector Concatenate/3  "<Re>"
  Bus Selector3/1 -> Vector Concatenate/4  "<Re>"

== system CAVE_MachE_speedTrack0202/Vehicle Under Test/Vehicle/Vehicle Dynamics/Vehicle 14DOF/Wheels and Tires/VDBS/Tires/Fiala Tires/alpha ==
  In1 : Inport
  In2 : Inport  Port=2
  In3 : Inport  Port=3
  In4 : Inport  Port=4
  Bus Selector{,1..3} (4 alike) : BusSelector  OutputSignals=Alpha
  Vector Concatenate : Concatenate  NumInputs=4
  Out1 : Outport  VectorParamsAs1DForOutWhenUnconnected=off
  wires:
  Vector Concatenate/1 -> Out1/1
  In1/1 -> Bus Selector/1
  Bus Selector/1 -> Vector Concatenate/1  "<Alpha>"
  In2/1 -> Bus Selector1/1
  In3/1 -> Bus Selector2/1
  In4/1 -> Bus Selector3/1
  Bus Selector1/1 -> Vector Concatenate/2  "<Alpha>"
  Bus Selector2/1 -> Vector Concatenate/3  "<Alpha>"
  Bus Selector3/1 -> Vector Concatenate/4  "<Alpha>"

== system CAVE_MachE_speedTrack0202/Vehicle Under Test/Vehicle/Vehicle Dynamics/Vehicle 14DOF/Wheels and Tires/VDBS/Tires/Fiala Tires/kappa ==
  In1 : Inport
  In2 : Inport  Port=2
  In3 : Inport  Port=3
  In4 : Inport  Port=4
  Bus Selector{,1..3} (4 alike) : BusSelector  OutputSignals=Kappa
  Vector Concatenate : Concatenate  NumInputs=4
  Out1 : Outport  VectorParamsAs1DForOutWhenUnconnected=off
  wires:
  Bus Selector3/1 -> Vector Concatenate/4  "<Kappa>"
  Bus Selector2/1 -> Vector Concatenate/3  "<Kappa>"
  Bus Selector1/1 -> Vector Concatenate/2  "<Kappa>"
  In4/1 -> Bus Selector3/1
  In3/1 -> Bus Selector2/1
  In2/1 -> Bus Selector1/1
  Bus Selector/1 -> Vector Concatenate/1  "<Kappa>"
  In1/1 -> Bus Selector/1
  Vector Concatenate/1 -> Out1/1

== system CAVE_MachE_speedTrack0202/Vehicle Under Test/Vehicle/Vehicle Dynamics/Vehicle 14DOF/Wheels and Tires/VDBS/Tires/Fiala Tires/omega ==
  In1 : Inport
  In2 : Inport  Port=2
  In3 : Inport  Port=3
  In4 : Inport  Port=4
  Bus Selector{,1..3} (4 alike) : BusSelector  OutputSignals=Omega
  Vector Concatenate : Concatenate  NumInputs=4
  Out1 : Outport  VectorParamsAs1DForOutWhenUnconnected=off
  wires:
  In1/1 -> Bus Selector/1
  Bus Selector/1 -> Vector Concatenate/1  "<Omega>"
  In2/1 -> Bus Selector1/1
  In3/1 -> Bus Selector2/1
  In4/1 -> Bus Selector3/1
  Bus Selector1/1 -> Vector Concatenate/2  "<Omega>"
  Bus Selector2/1 -> Vector Concatenate/3  "<Omega>"
  Bus Selector3/1 -> Vector Concatenate/4  "<Omega>"
  Vector Concatenate/1 -> Out1/1

== system CAVE_MachE_speedTrack0202/Vehicle Under Test/Vehicle/Vehicle Dynamics/Vehicle 14DOF/Wheels and Tires/VDBS/Tires/Fiala Tires/z ==
  In1 : Inport
  In2 : Inport  Port=2
  In3 : Inport  Port=3
  In4 : Inport  Port=4
  Bus Selector{,1..3} (4 alike) : BusSelector  OutputSignals=z
  Vector Concatenate : Concatenate  NumInputs=4
  Out1 : Outport  VectorParamsAs1DForOutWhenUnconnected=off
  wires:
  Bus Selector3/1 -> Vector Concatenate/4  "<z>"
  Bus Selector2/1 -> Vector Concatenate/3  "<z>"
  Bus Selector1/1 -> Vector Concatenate/2  "<z>"
  In4/1 -> Bus Selector3/1
  In3/1 -> Bus Selector2/1
  In2/1 -> Bus Selector1/1
  Bus Selector/1 -> Vector Concatenate/1  "<z>"
  In1/1 -> Bus Selector/1
  Vector Concatenate/1 -> Out1/1

== system CAVE_MachE_speedTrack0202/Vehicle Under Test/Vehicle/Vehicle Dynamics/Vehicle 14DOF/Wheels and Tires/VDBS/Tires/Fiala Tires/zdot ==
  In1 : Inport
  In2 : Inport  Port=2
  In3 : Inport  Port=3
  In4 : Inport  Port=4
  Bus Selector{,1..3} (4 alike) : BusSelector  OutputSignals=zdot
  Vector Concatenate : Concatenate  NumInputs=4
  Out1 : Outport  VectorParamsAs1DForOutWhenUnconnected=off
  wires:
  Vector Concatenate/1 -> Out1/1
  In1/1 -> Bus Selector/1
  Bus Selector/1 -> Vector Concatenate/1  "<zdot>"
  In2/1 -> Bus Selector1/1
  In3/1 -> Bus Selector2/1
  In4/1 -> Bus Selector3/1
  Bus Selector1/1 -> Vector Concatenate/2  "<zdot>"
  Bus Selector2/1 -> Vector Concatenate/3  "<zdot>"
  Bus Selector3/1 -> Vector Concatenate/4  "<zdot>"

== system CAVE_MachE_speedTrack0202/Vehicle Under Test/Vehicle/Vehicle Dynamics/Vehicle 14DOF/Wheels and Tires/VDBS/Tires/MF Tires/Fx ==
  In1 : Inport
  In2 : Inport  Port=2
  In3 : Inport  Port=3
  In4 : Inport  Port=4
  Bus Selector{,1..3} (4 alike) : BusSelector  OutputSignals=Fx
  Vector Concatenate : Concatenate  NumInputs=4
  Out1 : Outport  VectorParamsAs1DForOutWhenUnconnected=off
  wires:
  Bus Selector3/1 -> Vector Concatenate/4  "<Fx>"
  Bus Selector2/1 -> Vector Concatenate/3  "<Fx>"
  Bus Selector1/1 -> Vector Concatenate/2  "<Fx>"
  In4/1 -> Bus Selector3/1
  In3/1 -> Bus Selector2/1
  In2/1 -> Bus Selector1/1
  Bus Selector/1 -> Vector Concatenate/1  "<Fx>"
  In1/1 -> Bus Selector/1
  Vector Concatenate/1 -> Out1/1

== system CAVE_MachE_speedTrack0202/Vehicle Under Test/Vehicle/Vehicle Dynamics/Vehicle 14DOF/Wheels and Tires/VDBS/Tires/MF Tires/Fy ==
  In1 : Inport
  In2 : Inport  Port=2
  In3 : Inport  Port=3
  In4 : Inport  Port=4
  Bus Selector{,1..3} (4 alike) : BusSelector  OutputSignals=Fy
  Vector Concatenate : Concatenate  NumInputs=4
  Out1 : Outport  VectorParamsAs1DForOutWhenUnconnected=off
  wires:
  Vector Concatenate/1 -> Out1/1
  In1/1 -> Bus Selector/1
  Bus Selector/1 -> Vector Concatenate/1  "<Fy>"
  In2/1 -> Bus Selector1/1
  In3/1 -> Bus Selector2/1
  In4/1 -> Bus Selector3/1
  Bus Selector1/1 -> Vector Concatenate/2  "<Fy>"
  Bus Selector2/1 -> Vector Concatenate/3  "<Fy>"
  Bus Selector3/1 -> Vector Concatenate/4  "<Fy>"

== system CAVE_MachE_speedTrack0202/Vehicle Under Test/Vehicle/Vehicle Dynamics/Vehicle 14DOF/Wheels and Tires/VDBS/Tires/MF Tires/Fz ==
  In1 : Inport
  In2 : Inport  Port=2
  In3 : Inport  Port=3
  In4 : Inport  Port=4
  Bus Selector{,1..3} (4 alike) : BusSelector  OutputSignals=Fz
  Vector Concatenate : Concatenate  NumInputs=4
  Out1 : Outport  VectorParamsAs1DForOutWhenUnconnected=off
  wires:
  Vector Concatenate/1 -> Out1/1
  In1/1 -> Bus Selector/1
  Bus Selector/1 -> Vector Concatenate/1  "<Fz>"
  In2/1 -> Bus Selector1/1
  In3/1 -> Bus Selector2/1
  In4/1 -> Bus Selector3/1
  Bus Selector1/1 -> Vector Concatenate/2  "<Fz>"
  Bus Selector2/1 -> Vector Concatenate/3  "<Fz>"
  Bus Selector3/1 -> Vector Concatenate/4  "<Fz>"

== system CAVE_MachE_speedTrack0202/Vehicle Under Test/Vehicle/Vehicle Dynamics/Vehicle 14DOF/Wheels and Tires/VDBS/Tires/MF Tires/Mx ==
  In1 : Inport
  In2 : Inport  Port=2
  In3 : Inport  Port=3
  In4 : Inport  Port=4
  Bus Selector{,1..3} (4 alike) : BusSelector  OutputSignals=Mx
  Vector Concatenate : Concatenate  NumInputs=4
  Out1 : Outport  VectorParamsAs1DForOutWhenUnconnected=off
  wires:
  Vector Concatenate/1 -> Out1/1
  In1/1 -> Bus Selector/1
  Bus Selector/1 -> Vector Concatenate/1  "<Mx>"
  In2/1 -> Bus Selector1/1
  In3/1 -> Bus Selector2/1
  In4/1 -> Bus Selector3/1
  Bus Selector1/1 -> Vector Concatenate/2  "<Mx>"
  Bus Selector2/1 -> Vector Concatenate/3  "<Mx>"
  Bus Selector3/1 -> Vector Concatenate/4  "<Mx>"

== system CAVE_MachE_speedTrack0202/Vehicle Under Test/Vehicle/Vehicle Dynamics/Vehicle 14DOF/Wheels and Tires/VDBS/Tires/MF Tires/My ==
  In1 : Inport
  In2 : Inport  Port=2
  In3 : Inport  Port=3
  In4 : Inport  Port=4
  Bus Selector{,1..3} (4 alike) : BusSelector  OutputSignals=My
  Vector Concatenate : Concatenate  NumInputs=4
  Out1 : Outport  VectorParamsAs1DForOutWhenUnconnected=off
  wires:
  Bus Selector3/1 -> Vector Concatenate/4  "<My>"
  Bus Selector2/1 -> Vector Concatenate/3  "<My>"
  Bus Selector1/1 -> Vector Concatenate/2  "<My>"
  In4/1 -> Bus Selector3/1
  In3/1 -> Bus Selector2/1
  In2/1 -> Bus Selector1/1
  Bus Selector/1 -> Vector Concatenate/1  "<My>"
  In1/1 -> Bus Selector/1
  Vector Concatenate/1 -> Out1/1

== system CAVE_MachE_speedTrack0202/Vehicle Under Test/Vehicle/Vehicle Dynamics/Vehicle 14DOF/Wheels and Tires/VDBS/Tires/MF Tires/Mz ==
  In1 : Inport
  In2 : Inport  Port=2
  In3 : Inport  Port=3
  In4 : Inport  Port=4
  Bus Selector{,1..3} (4 alike) : BusSelector  OutputSignals=Mz
  Vector Concatenate : Concatenate  NumInputs=4
  Out1 : Outport  VectorParamsAs1DForOutWhenUnconnected=off
  wires:
  Bus Selector3/1 -> Vector Concatenate/4  "<Mz>"
  Bus Selector2/1 -> Vector Concatenate/3  "<Mz>"
  Bus Selector1/1 -> Vector Concatenate/2  "<Mz>"
  In4/1 -> Bus Selector3/1
  In3/1 -> Bus Selector2/1
  In2/1 -> Bus Selector1/1
  Bus Selector/1 -> Vector Concatenate/1  "<Mz>"
  In1/1 -> Bus Selector/1
  Vector Concatenate/1 -> Out1/1

== system CAVE_MachE_speedTrack0202/Vehicle Under Test/Vehicle/Vehicle Dynamics/Vehicle 14DOF/Wheels and Tires/VDBS/Tires/MF Tires/Re ==
  In1 : Inport
  In2 : Inport  Port=2
  In3 : Inport  Port=3
  In4 : Inport  Port=4
  Bus Selector{,1..3} (4 alike) : BusSelector  OutputSignals=Re
  Vector Concatenate : Concatenate  NumInputs=4
  Out1 : Outport  VectorParamsAs1DForOutWhenUnconnected=off
  wires:
  Vector Concatenate/1 -> Out1/1
  In1/1 -> Bus Selector/1
  Bus Selector/1 -> Vector Concatenate/1  "<Re>"
  In2/1 -> Bus Selector1/1
  In3/1 -> Bus Selector2/1
  In4/1 -> Bus Selector3/1
  Bus Selector1/1 -> Vector Concatenate/2  "<Re>"
  Bus Selector2/1 -> Vector Concatenate/3  "<Re>"
  Bus Selector3/1 -> Vector Concatenate/4  "<Re>"

== system CAVE_MachE_speedTrack0202/Vehicle Under Test/Vehicle/Vehicle Dynamics/Vehicle 14DOF/Wheels and Tires/VDBS/Tires/MF Tires/alpha ==
  In1 : Inport
  In2 : Inport  Port=2
  In3 : Inport  Port=3
  In4 : Inport  Port=4
  Bus Selector{,1..3} (4 alike) : BusSelector  OutputSignals=Alpha
  Vector Concatenate : Concatenate  NumInputs=4
  Out1 : Outport  VectorParamsAs1DForOutWhenUnconnected=off
  wires:
  Vector Concatenate/1 -> Out1/1
  In1/1 -> Bus Selector/1
  Bus Selector/1 -> Vector Concatenate/1  "<Alpha>"
  In2/1 -> Bus Selector1/1
  In3/1 -> Bus Selector2/1
  In4/1 -> Bus Selector3/1
  Bus Selector1/1 -> Vector Concatenate/2  "<Alpha>"
  Bus Selector2/1 -> Vector Concatenate/3  "<Alpha>"
  Bus Selector3/1 -> Vector Concatenate/4  "<Alpha>"

== system CAVE_MachE_speedTrack0202/Vehicle Under Test/Vehicle/Vehicle Dynamics/Vehicle 14DOF/Wheels and Tires/VDBS/Tires/MF Tires/kappa ==
  In1 : Inport
  In2 : Inport  Port=2
  In3 : Inport  Port=3
  In4 : Inport  Port=4
  Bus Selector{,1..3} (4 alike) : BusSelector  OutputSignals=Kappa
  Vector Concatenate : Concatenate  NumInputs=4
  Out1 : Outport  VectorParamsAs1DForOutWhenUnconnected=off
  wires:
  Bus Selector3/1 -> Vector Concatenate/4  "<Kappa>"
  Bus Selector2/1 -> Vector Concatenate/3  "<Kappa>"
  Bus Selector1/1 -> Vector Concatenate/2  "<Kappa>"
  In4/1 -> Bus Selector3/1
  In3/1 -> Bus Selector2/1
  In2/1 -> Bus Selector1/1
  Bus Selector/1 -> Vector Concatenate/1  "<Kappa>"
  In1/1 -> Bus Selector/1
  Vector Concatenate/1 -> Out1/1

== system CAVE_MachE_speedTrack0202/Vehicle Under Test/Vehicle/Vehicle Dynamics/Vehicle 14DOF/Wheels and Tires/VDBS/Tires/MF Tires/omega ==
  In1 : Inport
  In2 : Inport  Port=2
  In3 : Inport  Port=3
  In4 : Inport  Port=4
  Abs{,1..3} (4 alike) : Abs
  Bus Selector{,1..3} (4 alike) : BusSelector  OutputSignals=Omega
  Constant : Constant  Value=0
  Rate Limiter{,1..3} (4 alike) : RateLimiter  RisingSlewLimit=3  FallingSlewLimit=-3  SampleTimeMode=inherited
  Switch{1..4} (4 alike) : Switch  Criteria=u2 > Threshold  Threshold=0.11
  Transfer Fcn{,1..3} (4 alike) : TransferFcn  Denominator=[0.1 1]
  Vector Concatenate : Concatenate  NumInputs=4
  Out1 : Outport  VectorParamsAs1DForOutWhenUnconnected=off
  wires:
  In1/1 -> Bus Selector/1
  In2/1 -> Bus Selector1/1
  In3/1 -> Bus Selector2/1
  In4/1 -> Bus Selector3/1
  Vector Concatenate/1 -> Out1/1
  Abs2/1 -> Switch3/2
  Switch3/1 -> Vector Concatenate/3
  Bus Selector3/1 -> Rate Limiter3/1  "<Omega>"
  Rate Limiter1/1 -> Transfer Fcn1/1
  Rate Limiter2/1 -> Transfer Fcn2/1
  Bus Selector2/1 -> Rate Limiter2/1  "<Omega>"
  Bus Selector/1 -> Rate Limiter/1  "<Omega>"
  Switch4/1 -> Vector Concatenate/4
  Switch2/1 -> Vector Concatenate/2
  Rate Limiter/1 -> Transfer Fcn/1
  Transfer Fcn3/1 -> Abs3/1, Switch4/1
  Transfer Fcn1/1 -> Abs1/1, Switch2/1
  Constant/1 -> Switch4/3, Switch3/3, Switch2/3, Switch1/3
  Abs3/1 -> Switch4/2
  Switch1/1 -> Vector Concatenate/1
  Abs/1 -> Switch1/2
  Abs1/1 -> Switch2/2
  Transfer Fcn2/1 -> Abs2/1, Switch3/1
  Rate Limiter3/1 -> Transfer Fcn3/1
  Bus Selector1/1 -> Rate Limiter1/1  "<Omega>"
  Transfer Fcn/1 -> Switch1/1, Abs/1

== system CAVE_MachE_speedTrack0202/Vehicle Under Test/Vehicle/Vehicle Dynamics/Vehicle 14DOF/Wheels and Tires/VDBS/Tires/MF Tires/omega1 ==
  In1 : Inport
  In2 : Inport  Port=2
  In3 : Inport  Port=3
  In4 : Inport  Port=4
  Abs{,1..3} (4 alike) : Abs
  Constant : Constant  Value=0
  Rate Limiter{,1..3} (4 alike) : RateLimiter  RisingSlewLimit=5  FallingSlewLimit=-5  SampleTimeMode=inherited
  Switch{1..4} (4 alike) : Switch  Criteria=u2 > Threshold  Threshold=0.11
  Transfer Fcn{,1..3} (4 alike) : TransferFcn  Denominator=[0.1 1]
  Vector Concatenate : Concatenate  NumInputs=4
  Out1 : Outport  VectorParamsAs1DForOutWhenUnconnected=off
  wires:
  Vector Concatenate/1 -> Out1/1
  Abs2/1 -> Switch3/2
  Switch3/1 -> Vector Concatenate/3
  In4/1 -> Rate Limiter3/1
  Rate Limiter1/1 -> Transfer Fcn1/1
  Rate Limiter2/1 -> Transfer Fcn2/1
  In3/1 -> Rate Limiter2/1
  In1/1 -> Rate Limiter/1
  Switch4/1 -> Vector Concatenate/4
  Switch2/1 -> Vector Concatenate/2
  Rate Limiter/1 -> Transfer Fcn/1
  Transfer Fcn3/1 -> Abs3/1, Switch4/1
  Transfer Fcn1/1 -> Abs1/1, Switch2/1
  Constant/1 -> Switch4/3, Switch3/3, Switch2/3, Switch1/3
  Abs3/1 -> Switch4/2
  Switch1/1 -> Vector Concatenate/1
  Abs/1 -> Switch1/2
  Abs1/1 -> Switch2/2
  Transfer Fcn2/1 -> Abs2/1, Switch3/1
  Rate Limiter3/1 -> Transfer Fcn3/1
  In2/1 -> Rate Limiter1/1
  Transfer Fcn/1 -> Switch1/1, Abs/1

== system CAVE_MachE_speedTrack0202/Vehicle Under Test/Vehicle/Vehicle Dynamics/Vehicle 14DOF/Wheels and Tires/VDBS/Tires/MF Tires/z ==
  In1 : Inport
  In2 : Inport  Port=2
  In3 : Inport  Port=3
  In4 : Inport  Port=4
  Bus Selector{,1..3} (4 alike) : BusSelector  OutputSignals=z
  Vector Concatenate : Concatenate  NumInputs=4
  Out1 : Outport  VectorParamsAs1DForOutWhenUnconnected=off
  wires:
  Bus Selector3/1 -> Vector Concatenate/4  "<z>"
  Bus Selector2/1 -> Vector Concatenate/3  "<z>"
  Bus Selector1/1 -> Vector Concatenate/2  "<z>"
  In4/1 -> Bus Selector3/1
  In3/1 -> Bus Selector2/1
  In2/1 -> Bus Selector1/1
  Bus Selector/1 -> Vector Concatenate/1  "<z>"
  In1/1 -> Bus Selector/1
  Vector Concatenate/1 -> Out1/1

== system CAVE_MachE_speedTrack0202/Vehicle Under Test/Vehicle/Vehicle Dynamics/Vehicle 14DOF/Wheels and Tires/VDBS/Tires/MF Tires/zdot ==
  In1 : Inport
  In2 : Inport  Port=2
  In3 : Inport  Port=3
  In4 : Inport  Port=4
  Bus Selector{,1..3} (4 alike) : BusSelector  OutputSignals=zdot
  Vector Concatenate : Concatenate  NumInputs=4
  Out1 : Outport  VectorParamsAs1DForOutWhenUnconnected=off
  wires:
  Vector Concatenate/1 -> Out1/1
  In1/1 -> Bus Selector/1
  Bus Selector/1 -> Vector Concatenate/1  "<zdot>"
  In2/1 -> Bus Selector1/1
  In3/1 -> Bus Selector2/1
  In4/1 -> Bus Selector3/1
  Bus Selector1/1 -> Vector Concatenate/2  "<zdot>"
  Bus Selector2/1 -> Vector Concatenate/3  "<zdot>"
  Bus Selector3/1 -> Vector Concatenate/4  "<zdot>"

== matlab function CAVE_MachE_speedTrack0202/Vehicle Under Test/Vehicle/Vehicle Dynamics/Vehicle 7DOF/For 3D Visualization ==
  data: angles output size=3; angleIn input size=3; GeomXYZ output size=3; GemoXYZIn input size=3; GroundZ input size=4; trackW parameter; wheelB parameter
function [angles,GeomXYZ]= three26(angleIn, GemoXYZIn, GroundZ,trackW, wheelB)%#codegen
coder.allowpcode('plain')
% Copyright 2018 The MathWorks, Inc.
[angles,GeomXYZ]= vdynthree2six(angleIn, GemoXYZIn, GroundZ,trackW, wheelB);
